simulink model "pwr_amp_2x"  (Simulink 7.4)
settings: Solver=ode23tb  StartTime=0.0  StopTime=.012  MaxStep=1/(4*1e6)  RelTol=1e-3
PreLoadFcn:
  | R=8;      % load resistance
  | fc=80e3;  % bandpass corner
  | 
  | w=2*pi*fc;
  | 
  | c1=1.5012; l2=0.978; c3=.612;l4=.211;  % Rs=inf,  Rl = 1
  | % scale for freq and impedance ...
  | C1=c1/(R*w);
  | L2=l2*R/w;
  | C3=c3/(R*w);
  | L4=l4*R/w;
undefined symbols (not defined in the file or in its folder): C1, One, sided
libraries: powerlib x21, simulink x2, dspsnks4 x1, dsparch4 x1, simulink_extras x1
settings Model: Creator=dbenson  LastModifiedBy=Dick
settings SolverCC: InitialStep=1e-9  ZeroCrossControl=EnableAll  SolverResetMethod=Robust
settings DataIOCC: LimitDataPoints=off  SaveOutput=off  SaveTime=off  SignalLoggingName=sigsOut
settings OptimizationCC: BooleanDataType=off  InlineInvariantSignals=on  InitFltsAndDblsToZero=on
settings DebuggingCC: SaveWithParameterizedLinksMsg=none  SignalResolutionControl=TryResolveAllWithWarning  SolverPrmCheckMsg=none  MultiTaskDSMMsg=warning  MultiTaskCondExecSysMsg=none  StrictBusMsg=None
settings HardwareCC: TargetUnknown=on
settings RTWCC: IncludeERTFirstTime=on
settings GRTTargetCC: TargetFcnLib=ansi_tfl_tmw.mat

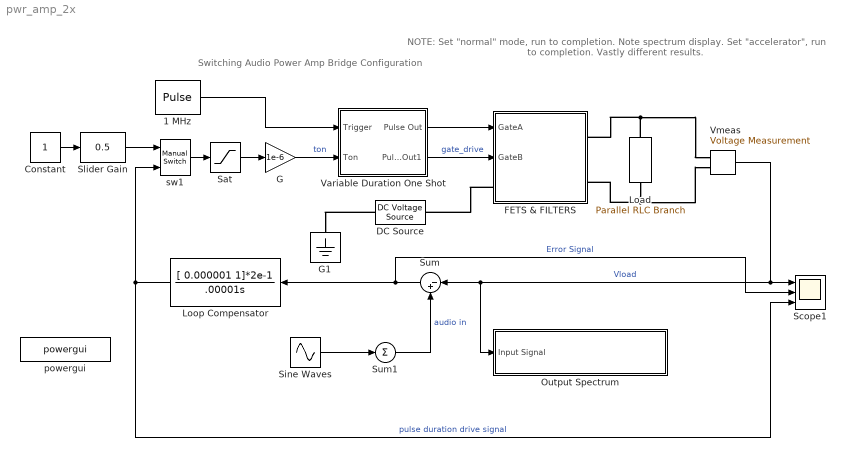
== system pwr_amp_2x ==
  note: Switching Audio Power Amp
      | Bridge Configuration
  note: NOTE: Set "normal" mode, run to completion. Note spectrum display.
      | Set "accelerator", run to completion. Vastly different results.
  1 MHz : DiscretePulseGenerator  PulseType=Time based  Amplitude=1  Period=1/1e6;  PulseWidth=50  PhaseDelay=.5e-6  SampleTime=1
  Constant : Constant  OutDataType=sfix(16)  OutScaling=2^0
  DC Source : powerlib/Electrical Sources/DC Voltage Source  Description=source block  DialogController=POWERSYS.PowerSysDialog  SystemSampleTime=-1  Amplitude=30  Measurements=None
      settings: AttributesFormatString=\n
  FETS & FILTERS : Subsystem
  G : Gain  Gain=1e-6  ParameterDataType=sfix(16)  ParameterScaling=2^0  OutDataType=sfix(16)  OutScaling=2^0  SaturateOnIntegerOverflow=on  OutDataTypeStr=Inherit: Same as input  ParamDataTypeStr=Inherit: Same as input
  G1 : powerlib/Elements/Ground  DialogController=POWERSYS.PowerSysDialog  PhysicalDomain=powersysdomain  SubClassName=unknown  LeftPortType=p1  RightPortType=p1  LConnTagsString=a
  Load : powerlib/Elements/Parallel RLC Branch  DialogController=POWERSYS.PowerSysDialog  PhysicalDomain=powersysdomain  SubClassName=unknown  LeftPortType=p1  RightPortType=p1  LConnTagsString=a  RConnTagsString=__new0  BranchType=R  Resistance=8  Inductance=1.0  SetiL0=off  InitialCurrent=0  Capacitance=1.0  Setx0=off  InitialVoltage=0  Measurements=None
  Loop Compensator : TransferFcn  Numerator=[ 0.000001 1]*2e-1  Denominator=[.00001 0]
  Output Spectrum : Subsystem  Description=Spectrum Analyzer  mask{BW=20e3, Zo=8}
      mask prompts: BW "Bandwidth"; Zo "Load Zo"
      mask Display: fprintf('Baseband Spectrum Analyzer \n  BW=%7.2f MHz', BW/1e6)
  Sat : Saturate  UpperLimit=0.95  LowerLimit=.01
  Scope1 : Scope  NumInputPorts=3
      settings: TimeRange=0.025  YMin=-20~-0.5786666666666638~0  YMax=20~0.5832888888888896~1  SaveName=ScopeData2  MaxDataPoints=50000  Decimation=100
  Sine Waves : Sin  Amplitude=10  Bias=0  Frequency=2*pi*[2000,2500]  Phase=0  Samples=10  SampleTime=0  Offset=0
  Slider Gain : simulink/Math Operations/Slider Gain  SystemSampleTime=-1  low=0  gain=0.5  high=1
  Sum : Sum  Inputs=|-+  OutDataType=sfix(16)  OutScaling=2^0  SaturateOnIntegerOverflow=on  InputSameDT=on  OutDataTypeStr=Inherit: Same as first input
  Sum1 : Sum  Inputs=+  OutDataType=sfix(16)  OutScaling=2^0
  Variable Duration One Shot : Subsystem
  Vmeas : powerlib/Measurements/Voltage Measurement  Tag=PoWeRsYsTeMmEaSuReMeNt  DialogController=POWERSYS.PowerSysDialog  SystemSampleTime=-1  PhasorSimulation=off  OutputType=Magnitude  PSBequivalent=0
  powergui : powerlib/powergui  SystemSampleTime=-1  SimulationMode=Continuous  SampleTime=50e-6  frequency=60  SPID=off  DisableSnubberDevices=off  DisableRonSwitches=off  DisableVfSwitches=off  SwTol=0  Interpol=off  frequencyindice=0  echomessages=off  HookPort=off  DisplayEquations=off  FunctionMessages=off  EnableUseOfTLC=off  x0status=blocks  RestoreLinks=warning  Frange=[0:2:500]  Ylog=off  Xlog=on  ShowGrid=off  save=off  variable=ZData  ZoomFFT=on  StartTime=0.0  cycles=1  DisplayStyle=1  fundamental=60  FreqAxis=off  MaxFrequency=1000  frequencyindicesteady=1  RmsSteady=1  display=off  Ts=0  methode=off
  sw1 : simulink/Signal Routing/Manual Switch  SystemSampleTime=-1  sw=0  action=0  varsize=off
  wires:
  1 MHz/1 -> Variable Duration One Shot/1(Trigger)
  Sum/1 -> Scope1/2, Loop Compensator/1  "Error Signal"
  G/1 -> Variable Duration One Shot/2(Ton)  "ton"
  Sat/1 -> G/1
  sw1/1 -> Sat/1
  Constant/1 -> Slider Gain/1
  Slider Gain/1 -> sw1/1
  Sine Waves/1 -> Sum1/1
  Sum1/1 -> Sum/2  "audio in"
  Variable Duration One Shot/1(Pulse Out) -> FETS & FILTERS/1(GateA)
  Variable Duration One Shot/2(Pulse Out1) -> FETS & FILTERS/2(GateB)  "gate_drive"
  Vmeas/1 -> Scope1/1, Sum/1, Output Spectrum/1(Input Signal)  "Vload"
  Loop Compensator/1 -> sw1/2, Scope1/3  "pulse duration drive signal"
  connections:
  DC Source/LConn1 -- G1/LConn1
  FETS & FILTERS/LConn1 -- DC Source/RConn1
  Load/RConn1 -- FETS & FILTERS/RConn1 -- Vmeas/LConn1
  Load/LConn1 -- FETS & FILTERS/RConn2 -- Vmeas/LConn2

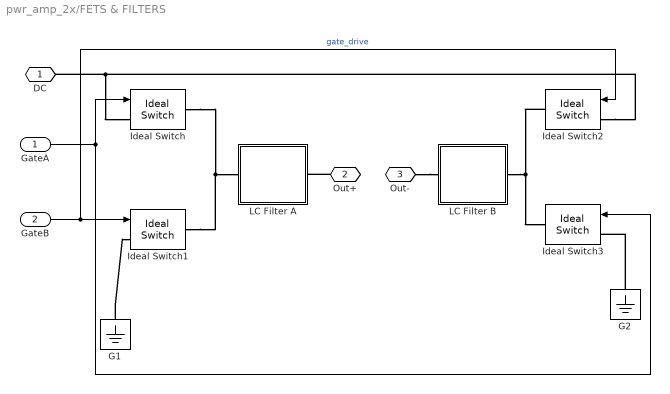
== system pwr_amp_2x/FETS & FILTERS ==
  GateA : Inport  OutDataType=sfix(16)  OutScaling=2^0
  GateB : Inport  Port=2  OutDataType=sfix(16)  OutScaling=2^0
  G1 : powerlib/Elements/Ground  DialogController=POWERSYS.PowerSysDialog  PhysicalDomain=powersysdomain  SubClassName=unknown  LeftPortType=p1  RightPortType=p1  LConnTagsString=a
  G2 : powerlib/Elements/Ground  DialogController=POWERSYS.PowerSysDialog  PhysicalDomain=powersysdomain  SubClassName=unknown  LeftPortType=p1  RightPortType=p1  LConnTagsString=a
  Ideal Switch{,1..3} (4 alike) : powerlib/Power Electronics/Ideal Switch  DialogController=POWERSYS.PowerSysDialog  SystemSampleTime=-1  Ron=0.1  Lon=0  IC=0  Rs=0  Cs=0  Measurements=off
      settings: AttributesFormatString=\n
  LC Filter A : Subsystem
  LC Filter B : Subsystem
  DC : PMIOPort  Port=1  Side=Left
  Out+ : PMIOPort  Port=2  Side=Right
  Out- : PMIOPort  Port=3  Side=Right
  wires:
  GateA/1 -> Ideal Switch3/1, Ideal Switch/1
  GateB/1 -> Ideal Switch2/1, Ideal Switch1/1  "gate_drive"
  connections:
  DC/RConn1 -- Ideal Switch2/LConn1 -- Ideal Switch/LConn1
  Ideal Switch2/RConn1 -- LC Filter B/LConn1 -- Ideal Switch3/RConn1
  Out+/RConn1 -- LC Filter A/RConn1
  Ideal Switch/RConn1 -- LC Filter A/LConn1 -- Ideal Switch1/RConn1
  Out-/RConn1 -- LC Filter B/RConn1
  G1/LConn1 -- Ideal Switch1/LConn1
  G2/LConn1 -- Ideal Switch3/LConn1

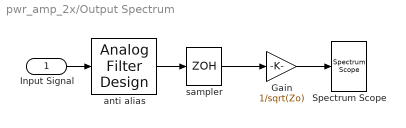
== system pwr_amp_2x/Output Spectrum ==
  Input Signal : Inport  OutDataType=sfix(16)  OutScaling=2^0
  Gain : Gain  Gain=1/sqrt(Zo)  ParameterDataType=fixdt(1, 16)  ParameterScaling=2^0  OutDataType=fixdt(1, 16)  OutScaling=2^0
  Spectrum Scope : dspsnks4/Spectrum Scope  DialogController=dspdialog.SpectrumScope  DialogControllerArgs=DataTag0  SystemSampleTime=-1  ScopeProperties=on  Domain=Frequency  HorizSpan=1  UseBuffer=on  BufferSize=512  Overlap=0  inpFftLenInherit=off  FFTlength=128  numAvg=1  DisplayProperties=off  AxisGrid=on  Memory=off  FrameNumber=on  AxisLegend=off  AxisZoom=off  OpenScopeAtSimStart=on  OpenScopeImmediately=off  FigPos=[438 61 408 280]  AxisProperties=off  XUnits=Hertz  XRange=One-sided ([0...Fs/2])  XDisplay=0  InheritXIncr=on  XIncr=1.0  XLabel=Samples  XLimit=Auto  YUnits=dBW  XMax=1  XMin=0  YLabel=dBW  LineProperties=off  wintypeSpecScope=Hann  RsSpecScope=50  betaSpecScope=5  winsampSpecScope=Periodic  XAxisParamsVer=6.9
      settings: YMin=-100  YMax=10
  anti alias : dsparch4/Analog Filter Design  method=Elliptic  filttype=Lowpass  N=8  Wlo=BW*2*pi  Whi=80  Rp=0.11  Rs=100
  sampler : ZeroOrderHold  SampleTime=1/(2.56*BW)
  wires:
  Gain/1 -> Spectrum Scope/1
  Input Signal/1 -> anti alias/1
  anti alias/1 -> sampler/1
  sampler/1 -> Gain/1

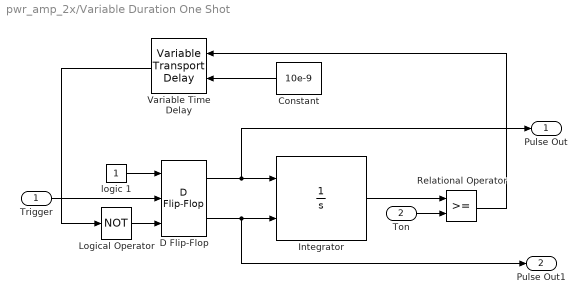
== system pwr_amp_2x/Variable Duration One Shot ==
  Trigger : Inport  OutDataType=sfix(16)  OutScaling=2^0
  Ton : Inport  Port=2  OutDataType=sfix(16)  OutScaling=2^0
  Constant : Constant  Value=10e-9  OutDataType=fixdt(1, 16)  OutScaling=2^0
  D Flip-Flop : simulink_extras/Flip Flops/D Flip-Flop  SystemSampleTime=-1
  Integrator : Integrator  ExternalReset=level
  Logical Operator : Logic  Operator=NOT
  Relational Operator : RelationalOperator  InputSameDT=on
  Variable Time Delay : VariableTransportDelay  MaximumDelay=20e-9  MaximumPoints=2^12  FixedBuffer=on
  logic 1 : Constant  OutDataType=sfix(16)  OutScaling=2^0
  Pulse Out : Outport  OutDataType=sfix(16)  OutScaling=2^0
  Pulse Out1 : Outport  Port=2  OutDataType=sfix(16)  OutScaling=2^0
  wires:
  D Flip-Flop/2 -> Integrator/2, Pulse Out1/1
  logic 1/1 -> D Flip-Flop/1
  Logical Operator/1 -> D Flip-Flop/3
  Integrator/1 -> Relational Operator/1
  D Flip-Flop/1 -> Integrator/1, Pulse Out/1
  Trigger/1 -> D Flip-Flop/2
  Ton/1 -> Relational Operator/2
  Constant/1 -> Variable Time Delay/2
  Variable Time Delay/1 -> Logical Operator/1
  Relational Operator/1 -> Variable Time Delay/1

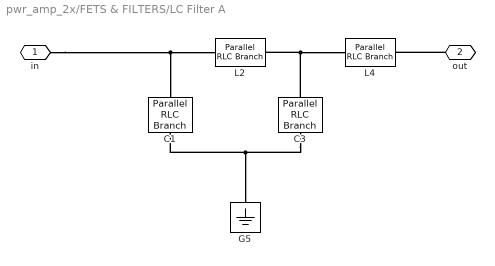
== system pwr_amp_2x/FETS & FILTERS/LC Filter A ==
  C1 : powerlib/Elements/Parallel RLC Branch  DialogController=POWERSYS.PowerSysDialog  PhysicalDomain=powersysdomain  SubClassName=unknown  LeftPortType=p1  RightPortType=p1  LConnTagsString=a  RConnTagsString=__new0  BranchType=C  Resistance=1.0  Inductance=1.0  SetiL0=off  InitialCurrent=0  Capacitance=C1  Setx0=off  InitialVoltage=0  Measurements=None
  C3 : powerlib/Elements/Parallel RLC Branch  DialogController=POWERSYS.PowerSysDialog  PhysicalDomain=powersysdomain  SubClassName=unknown  LeftPortType=p1  RightPortType=p1  LConnTagsString=a  RConnTagsString=__new0  BranchType=C  Resistance=1.0  Inductance=1.0  SetiL0=off  InitialCurrent=0  Capacitance=C3  Setx0=off  InitialVoltage=0  Measurements=None
  G5 : powerlib/Elements/Ground  DialogController=POWERSYS.PowerSysDialog  PhysicalDomain=powersysdomain  SubClassName=unknown  LeftPortType=p1  RightPortType=p1  LConnTagsString=a
  L2 : powerlib/Elements/Parallel RLC Branch  DialogController=POWERSYS.PowerSysDialog  PhysicalDomain=powersysdomain  SubClassName=unknown  LeftPortType=p1  RightPortType=p1  LConnTagsString=a  RConnTagsString=__new0  BranchType=L  Resistance=1.0  Inductance=L2  SetiL0=off  InitialCurrent=0  Capacitance=1.0  Setx0=off  InitialVoltage=0  Measurements=None
  L4 : powerlib/Elements/Parallel RLC Branch  DialogController=POWERSYS.PowerSysDialog  PhysicalDomain=powersysdomain  SubClassName=unknown  LeftPortType=p1  RightPortType=p1  LConnTagsString=a  RConnTagsString=__new0  BranchType=L  Resistance=1.0  Inductance=L4  SetiL0=off  InitialCurrent=0  Capacitance=1.0  Setx0=off  InitialVoltage=0  Measurements=None
  in : PMIOPort  Port=1  Side=Left
  out : PMIOPort  Port=2  Side=Right
  connections:
  C3/LConn1 -- C1/LConn1 -- G5/LConn1
  C3/RConn1 -- L2/RConn1 -- L4/LConn1
  out/RConn1 -- L4/RConn1
  in/RConn1 -- C1/RConn1 -- L2/LConn1

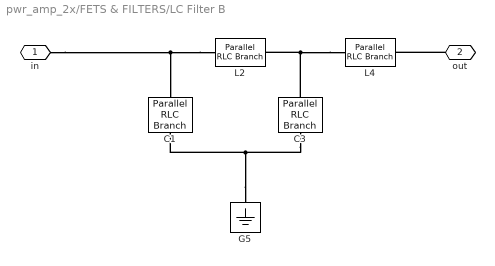
== system pwr_amp_2x/FETS & FILTERS/LC Filter B ==
  C1 : powerlib/Elements/Parallel RLC Branch  DialogController=POWERSYS.PowerSysDialog  PhysicalDomain=powersysdomain  SubClassName=unknown  LeftPortType=p1  RightPortType=p1  LConnTagsString=a  RConnTagsString=__new0  BranchType=C  Resistance=1.0  Inductance=1.0  SetiL0=off  InitialCurrent=0  Capacitance=C1  Setx0=off  InitialVoltage=0  Measurements=None
  C3 : powerlib/Elements/Parallel RLC Branch  DialogController=POWERSYS.PowerSysDialog  PhysicalDomain=powersysdomain  SubClassName=unknown  LeftPortType=p1  RightPortType=p1  LConnTagsString=a  RConnTagsString=__new0  BranchType=C  Resistance=1.0  Inductance=1.0  SetiL0=off  InitialCurrent=0  Capacitance=C3  Setx0=off  InitialVoltage=0  Measurements=None
  G5 : powerlib/Elements/Ground  DialogController=POWERSYS.PowerSysDialog  PhysicalDomain=powersysdomain  SubClassName=unknown  LeftPortType=p1  RightPortType=p1  LConnTagsString=a
  L2 : powerlib/Elements/Parallel RLC Branch  DialogController=POWERSYS.PowerSysDialog  PhysicalDomain=powersysdomain  SubClassName=unknown  LeftPortType=p1  RightPortType=p1  LConnTagsString=a  RConnTagsString=__new0  BranchType=L  Resistance=1.0  Inductance=L2  SetiL0=off  InitialCurrent=0  Capacitance=1.0  Setx0=off  InitialVoltage=0  Measurements=None
  L4 : powerlib/Elements/Parallel RLC Branch  DialogController=POWERSYS.PowerSysDialog  PhysicalDomain=powersysdomain  SubClassName=unknown  LeftPortType=p1  RightPortType=p1  LConnTagsString=a  RConnTagsString=__new0  BranchType=L  Resistance=1.0  Inductance=L4  SetiL0=off  InitialCurrent=0  Capacitance=1.0  Setx0=off  InitialVoltage=0  Measurements=None
  in : PMIOPort  Port=1  Side=Left
  out : PMIOPort  Port=2  Side=Right
  connections:
  L2/LConn1 -- C1/RConn1 -- in/RConn1
  out/RConn1 -- L4/RConn1
  L4/LConn1 -- L2/RConn1 -- C3/RConn1
  G5/LConn1 -- C1/LConn1 -- C3/LConn1
